simulink model "vector"  (R2022b)
settings: Solver=ode45  StartTime=0  StopTime=1  MaxStep=T_s  RelTol=1e-3  AbsTol=1e-3  EnableMultiTasking=on
values from neighbouring files (symbols this model uses):
  alpha_c = 2*pi*300    (= 1884.95559215)    [init_vector.m]    (also in task13.m; task13_2.m)
  alpha_s = 2*pi*20    (= 125.663706144)    [init_vector.m]
  J = 0.015    [init_vector.m]
  L_M = 0.224    [init_vector.m]    (also in task_4_script.m)
  L_sigma = 0.021    [init_vector.m]    (also in task_4_script.m)
  n_p = 2    [init_vector.m]
  psi_R_ref = 0.9    [init_vector.m]
  R_R = 2.1    [init_vector.m]
  T_s = 125e-6    (= 0.000125)    [init_vector.m]    (also in init_vhz.m; task13_2.m)
  tau_M_max = 20    [init_vector.m]
libraries: simulink x1
settings Model: Creator=mhinkkan  LastModifiedBy=mhinkkan
settings SolverCC: AutoScaleAbsTol=off  AlgebraicLoopSolver=TrustRegion
settings DataIOCC: SaveFormat=Array  SignalLoggingSaveFormat=ModelDataLogs  SaveOutput=off  SignalLogging=off  DSMLogging=off  SaveTime=off  ReturnWorkspaceOutputs=off
settings OptimizationCC: BlockReduction=off  BooleanDataType=off  DefaultParameterBehavior=Inlined  OptimizeBlockIOStorage=off  BufferReuse=off  GlobalBufferReuse=off  ExpressionFolding=off  ExpressionDepthLimit=2147483647  LocalBlockOutputs=off  InitFltsAndDblsToZero=on  LifeSpan=inf
settings DebuggingCC: SaveWithParameterizedLinksMsg=none  UnderspecifiedInitializationDetection=Classic  MergeDetectMultiDrivingBlocksExec=none  SignalResolutionControl=TryResolveAllWithWarning  MultiTaskDSMMsg=warning  MultiTaskCondExecSysMsg=none  FcnCallInpInsideContextMsg=warning  UnconnectedInputMsg=warning  UnconnectedOutputMsg=warning  UnconnectedLineMsg=warning  AllowSymbolicDim=off  StateNameClashWarn=warning  SFUnexpectedBacktrackingDiag=warning  SFNoUnconditionalDefaultTransitionDiag=warning  SFExecutionAtInitializationDiag=none  SFMachineParentedDataDiag=warning  ArithmeticOperatorsInVariantConditions=warning
settings HardwareCC: ProdBitPerPointer=32  ProdBitPerSizeT=32  ProdBitPerPtrDiffT=32  ProdLargestAtomicFloat=None  ProdIntDivRoundTo=Undefined  ProdEndianess=Unspecified  ProdWordSize=32  ProdHWDeviceType=32-bit Generic  TargetUnknown=on
settings ModelReferenceCC: EnableRefExpFcnMdlSchedulingChecks=on  PropagateSignalLabelsOutOfModel=off
settings SFSimCC: SimUseLocalCustomCode=off  CustomCodeUndefinedFunction=UseInterfaceOnly
settings RTWCC: RTWUseLocalCustomCode=off
settings CodeAppCC: StateflowObjectComments=on
settings GRTTargetCC: TargetFcnLib=ansi_tfl_tmw.mat  TargetLangStandard=C89/C90 (ANSI)  CombineOutputUpdateFcns=off  GRTInterface=on
settings ConfigComp: CovMetricSettings=dw  CovSaveCumulativeToWorkspaceVar=on  CovSaveSingleToWorkspaceVar=on  CovExternalEMLEnable=off

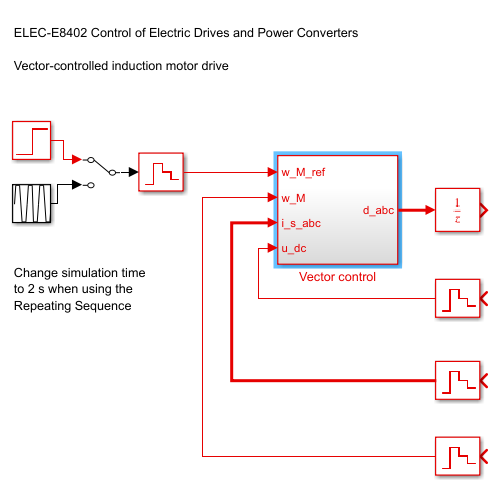
[thumbnail: Simulink's stored preview of the top-level diagram]
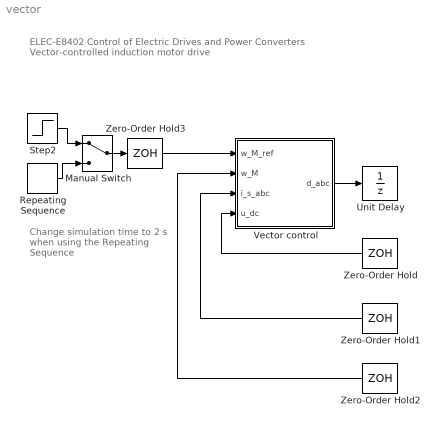
== system vector ==
  note: ELEC-E8402 Control of Electric Drives and Power Converters
      |
      | Vector-controlled induction motor drive
  note: Change simulation time
      | to 2 s when using the
      | Repeating Sequence
  Manual Switch : ManualSwitch
  Repeating Sequence : simulink/Sources/Repeating Sequence  rep_seq_t=[0 .2 .8 1.2 1.8 2]  rep_seq_y=2*pi*30/n_p*[0 1 1 -1 -1 0]
  Step2 : Step  Time=0.3  After=2*pi*40/n_p  SampleTime=T_s
  Unit Delay : UnitDelay  SampleTime=T_s  HasFrameUpgradeWarning=on
  Vector control : Subsystem
  Zero-Order Hold{,1..3} (4 alike) : ZeroOrderHold  SampleTime=T_s
  wires:
  Zero-Order Hold3/1 -> Vector control/1(w_M_ref)
  Zero-Order Hold/1 -> Vector control/4(u_dc)
  Zero-Order Hold1/1 -> Vector control/3(i_s_abc)
  Vector control/1(d_abc) -> Unit Delay/1
  Zero-Order Hold2/1 -> Vector control/2(w_M)
  Repeating Sequence/1 -> Manual Switch/2
  Step2/1 -> Manual Switch/1
  Manual Switch/1 -> Zero-Order Hold3/1

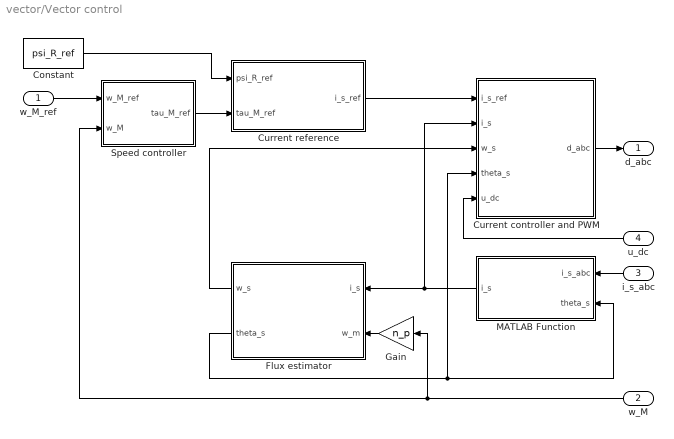
== system vector/Vector control ==
  w_M_ref : Inport
  w_M : Inport  Port=2
  i_s_abc : Inport  Port=3
  u_dc : Inport  Port=4
  Constant : Constant  Value=psi_R_ref  SampleTime=T_s
  Current controller and PWM : Subsystem
  Current reference : MATLAB Function  TreatAsAtomicUnit=on
  Flux estimator : Subsystem
  Gain : Gain  Gain=n_p  SaturateOnIntegerOverflow=on  OutDataTypeStr=Inherit: Same as input  ParamDataTypeStr=Inherit: Same as input
  MATLAB Function : MATLAB Function  TreatAsAtomicUnit=on
  Speed controller : Subsystem
  d_abc : Outport
  wires:
  Flux estimator/2(theta_s) -> Current controller and PWM/4(theta_s), MATLAB Function/2(theta_s)
  w_M/1 -> Gain/1, Speed controller/2(w_M)
  i_s_abc/1 -> MATLAB Function/1(i_s_abc)
  Current controller and PWM/1(d_abc) -> d_abc/1
  Current reference/1(i_s_ref) -> Current controller and PWM/1(i_s_ref)
  Flux estimator/1(w_s) -> Current controller and PWM/3(w_s)
  MATLAB Function/1(i_s) -> Current controller and PWM/2(i_s), Flux estimator/1(i_s)
  w_M_ref/1 -> Speed controller/1(w_M_ref)
  Constant/1 -> Current reference/1(psi_R_ref)
  u_dc/1 -> Current controller and PWM/5(u_dc)
  Speed controller/1(tau_M_ref) -> Current reference/2(tau_M_ref)
  Gain/1 -> Flux estimator/2(w_m)

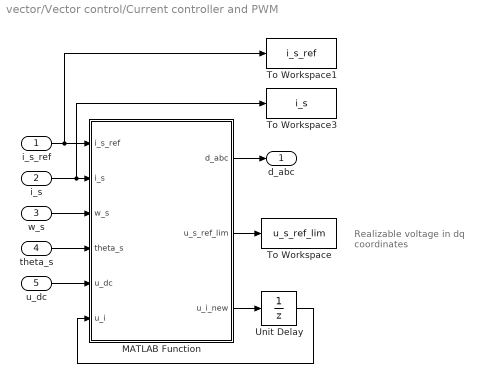
== system vector/Vector control/Current controller and PWM ==
  note: Realizable voltage
      | in dq coordinates
  i_s_ref : Inport
  i_s : Inport  Port=2
  w_s : Inport  Port=3
  theta_s : Inport  Port=4
  u_dc : Inport  Port=5
  MATLAB Function : MATLAB Function  TreatAsAtomicUnit=on
  To Workspace : ToWorkspace  VariableName=u_s_ref_lim  SaveFormat=Timeseries  SampleTime=-1
  To Workspace1 : ToWorkspace  VariableName=i_s_ref  SaveFormat=Timeseries  SampleTime=-1
  To Workspace3 : ToWorkspace  VariableName=i_s  SaveFormat=Timeseries  SampleTime=-1
  Unit Delay : UnitDelay  SampleTime=-1  HasFrameUpgradeWarning=on
  d_abc : Outport  PortDimensions=3
  wires:
  MATLAB Function/3(u_i_new) -> Unit Delay/1
  i_s_ref/1 -> To Workspace1/1, MATLAB Function/1(i_s_ref)
  w_s/1 -> MATLAB Function/3(w_s)
  i_s/1 -> To Workspace3/1, MATLAB Function/2(i_s)
  Unit Delay/1 -> MATLAB Function/6(u_i)
  theta_s/1 -> MATLAB Function/4(theta_s)
  u_dc/1 -> MATLAB Function/5(u_dc)
  MATLAB Function/1(d_abc) -> d_abc/1
  MATLAB Function/2(u_s_ref_lim) -> To Workspace/1

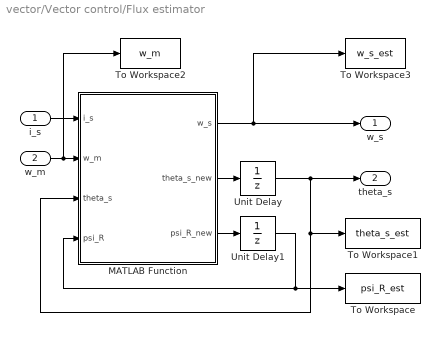
== system vector/Vector control/Flux estimator ==
  i_s : Inport
  w_m : Inport  Port=2
  MATLAB Function : MATLAB Function  TreatAsAtomicUnit=on
  To Workspace : ToWorkspace  VariableName=psi_R_est  SaveFormat=Timeseries  SampleTime=-1
  To Workspace1 : ToWorkspace  VariableName=theta_s_est  SaveFormat=Timeseries  SampleTime=-1
  To Workspace2 : ToWorkspace  VariableName=w_m  SaveFormat=Timeseries  SampleTime=-1
  To Workspace3 : ToWorkspace  VariableName=w_s_est  SaveFormat=Timeseries  SampleTime=-1
  Unit Delay : UnitDelay  SampleTime=-1  HasFrameUpgradeWarning=on
  Unit Delay1 : UnitDelay  SampleTime=-1  HasFrameUpgradeWarning=on
  w_s : Outport
  theta_s : Outport  Port=2
  wires:
  MATLAB Function/2(theta_s_new) -> Unit Delay/1
  MATLAB Function/1(w_s) -> To Workspace3/1, w_s/1
  w_m/1 -> To Workspace2/1, MATLAB Function/2(w_m)
  i_s/1 -> MATLAB Function/1(i_s)
  Unit Delay1/1 -> MATLAB Function/4(psi_R), To Workspace/1
  Unit Delay/1 -> MATLAB Function/3(theta_s), To Workspace1/1, theta_s/1
  MATLAB Function/3(psi_R_new) -> Unit Delay1/1

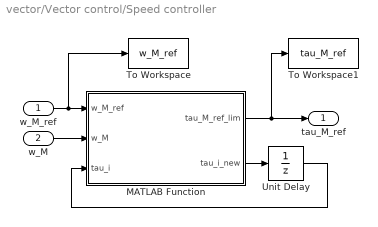
== system vector/Vector control/Speed controller ==
  w_M_ref : Inport
  w_M : Inport  Port=2
  MATLAB Function : MATLAB Function  TreatAsAtomicUnit=on
  To Workspace : ToWorkspace  VariableName=w_M_ref  SaveFormat=Timeseries  SampleTime=-1
  To Workspace1 : ToWorkspace  VariableName=tau_M_ref  SaveFormat=Timeseries  SampleTime=-1
  Unit Delay : UnitDelay  SampleTime=-1  HasFrameUpgradeWarning=on
  tau_M_ref : Outport
  wires:
  w_M_ref/1 -> To Workspace/1, MATLAB Function/1(w_M_ref)
  Unit Delay/1 -> MATLAB Function/3(tau_i)
  w_M/1 -> MATLAB Function/2(w_M)
  MATLAB Function/1(tau_M_ref_lim) -> To Workspace1/1, tau_M_ref/1
  MATLAB Function/2(tau_i_new) -> Unit Delay/1

== matlab function vector/Vector control/Current controller and PWM/MATLAB Function ==
  data: i_s_ref input size=1; i_s input size=1; w_s input size=1; theta_s input size=1; u_dc input size=1; u_i input size=1; L_sigma parameter size=1; alpha_c parameter size=1; T_s parameter size=1; d_abc output size=3; u_s_ref_lim output size=1; u_i_new output
function [d_abc, u_s_ref_lim, u_i_new] = cc(i_s_ref, i_s, w_s, theta_s, ...
    u_dc, u_i, L_sigma, alpha_c, T_s)

%% Current controller 
% Gains
k_i = alpha_c^2*L_sigma;                % Integral gain
k_t = alpha_c*L_sigma;                   % Reference gain
k_p = (2*alpha_c - 1j*w_s)*L_sigma;     % Proportional gain

% Voltage reference in synchronous coordinates
u_s_ref = k_t*i_s_ref - k_p*i_s + u_i;

% Reference in stator coordinates
theta_sc = theta_s + 1.5*T_s*w_s;   % Compensation for discrete-time delays
u_ss_ref = u_s_ref*exp(1j*theta_sc);

%% Symmetrical suboscillation PWM
% Components of the voltage space vector
u_alpha_ref = real(u_ss_ref);
u_beta_ref  = imag(u_ss_ref);

% Phase-voltage references
u_a_ref = u_alpha_ref;
u_b_ref = .5*(-u_alpha_ref + sqrt(3)*u_beta_ref);
u_c_ref = .5*(-u_alpha_ref - sqrt(3)*u_beta_ref);

% Vector of phase-voltage references
u_abc_ref = [u_a_ref; u_b_ref; u_c_ref];

% Symmetrization of the references by adding the zero-sequence voltage
u0 = .5*(max(u_abc_ref) + min(u_abc_ref));
u_abc_ref = u_abc_ref - u0;

% Clamping of the reference voltages such that no phase error is caused. 
% If all phase voltage reference are realizable (below Udc/2), m = 1 holds.
m = max([2*u_abc_ref/u_dc; 1]);
u_abc_ref = u_abc_ref/m;

% Duty cycles, which can be directly used for triangle comparison, 
% if the triangle wave varies between 0...1
d_abc = .5 + u_abc_ref/u_dc;

% Realized voltage vector is calculated from the clamped duty ratios.
% If the PWM does not saturate, us_ref_lim = us_ref holds. The realized
% voltage vector is needed, e.g., for the current-controller antiwindup.
u_ss_ref_lim = 2/3*(d_abc(1) + d_abc(2)*exp(1j*2*pi/3) ...
    + d_abc(3)*exp(1j*4*pi/3))*u_dc;
% In estimated rotor flux coordinates
u_s_ref_lim = exp(-1j*theta_sc)*u_ss_ref_lim;  

%% Update the integral state of the current controller 
u_i_new = u_i + T_s*k_i*(i_s_ref - i_s + (u_s_ref_lim - u_s_ref)/k_t);

== matlab function vector/Vector control/Flux estimator/MATLAB Function ==
  data: i_s input size=1; w_m input size=1; theta_s input size=1; psi_R input size=1; R_R parameter size=1; L_M parameter size=1; T_s parameter size=1; w_s output size=1; theta_s_new output size=1; psi_R_new output size=1
function [w_s, theta_s_new, psi_R_new] = estimator(i_s, w_m, theta_s, ...
    psi_R, R_R, L_M, T_s)

% Current components
i_d = real(i_s);
i_q = imag(i_s);

% Angular frequency of the rotor flux
if(psi_R > 0) 	                    % Avoid division by zero
	%w_s = ...;	                    % Complete this
else
	w_s = w_m;
end

% Update the states
%psi_R_new = ...;                	% Complete this
theta_s_new = theta_s + T_s*w_s;   	% Rotor flux angle

% Limit the angle between [-pi, pi]
while(theta_s_new > pi)
    theta_s_new = theta_s_new - 2*pi;
end
while(theta_s_new < -pi) 
    theta_s_new = theta_s_new + 2*pi;
end

== matlab function vector/Vector control/MATLAB Function ==
  data: i_s_abc input size=3; theta_s input size=1; i_s output size=1
function i_s = abc2dq(i_s_abc, theta_s)

% Phase currents
%i_a = i_s_abc(1); i_b = i_s_abc(2); i_c = i_s_abc(3); 

% Space-vector transformation and coordinate transformation
% i_s = ...		% Complete this

== matlab function vector/Vector control/Speed controller/MATLAB Function ==
  data: w_M_ref input size=1; w_M input size=1; tau_i input size=1; J parameter size=1; alpha_s parameter size=1; tau_M_max parameter size=1; tau_M_ref_lim output size=1; T_s parameter size=1; tau_i_new output
% 2DOF PI speed controller
function [tau_M_ref_lim, tau_i_new] = speed_ctrl(w_M_ref, w_M, tau_i, ...
    J, alpha_s, tau_M_max, T_s)

% Gains
k_i = alpha_s^2*J;
k_t = alpha_s*J;
k_p = 2*alpha_s*J;

% Ideal reference
tau_M_ref = k_t*w_M_ref - k_p*w_M + tau_i;

% Limited reference
tau_M_ref_lim = tau_M_ref;
if(tau_M_ref_lim > tau_M_max)
    tau_M_ref_lim = tau_M_max;
elseif(tau_M_ref_lim < -tau_M_max)
    tau_M_ref_lim = -tau_M_max;
end

% Update the integral state
tau_i_new = tau_i + T_s*k_i*(w_M_ref - w_M ...
    + (tau_M_ref_lim - tau_M_ref)/k_t);

== matlab function vector/Vector control/Current reference ==
  data: psi_R_ref input size=1; tau_M_ref input size=1; L_M parameter size=1; n_p parameter size=1; i_s_ref output size=1
function i_s_ref = curr_ref(psi_R_ref, tau_M_ref, L_M, n_p)

% Current reference in estimated rotor-flux coordinates
% i_d_ref = ...		% Complete this
% i_q_ref = ...		% Complete this
i_s_ref = i_d_ref + 1j*i_q_ref;
